simulink model "EPS Simulink Model"  (R2018b)
settings: Solver=VariableStepAuto  StartTime=0.0  StopTime=10.0  RelTol=1e-3
model workspace (MAT data in the model file):
  a = 4.4
  b = 2.25
settings Model: Creator=chaitu  LastModifiedBy=chaitu

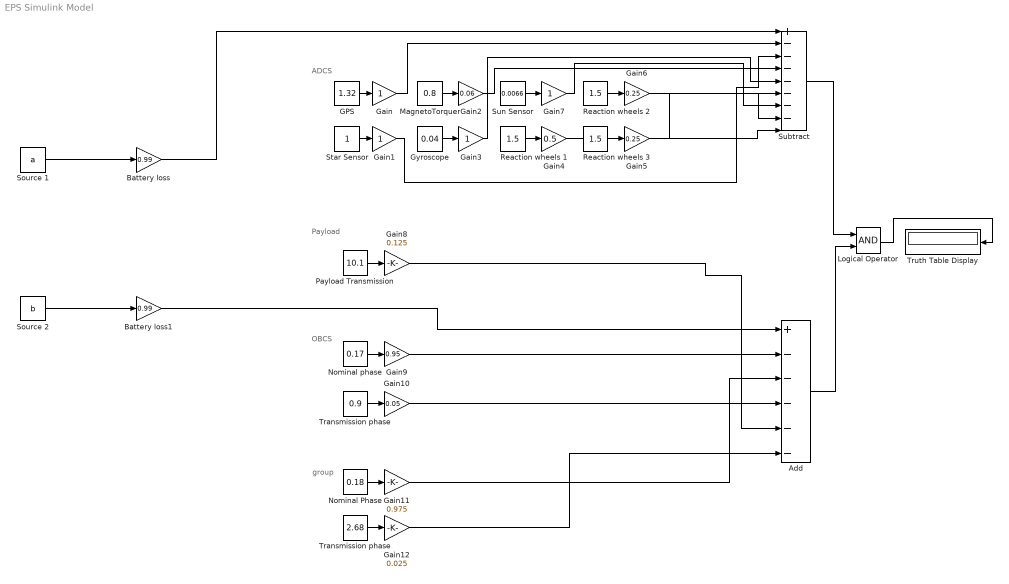
== system EPS Simulink Model ==
  note: group
  note: OBCS
  note: Payload
  note: ADCS
  Add : Sum  Inputs=+-----
  Battery loss : Gain  Gain=0.99
  Battery loss1 : Gain  Gain=0.99
  GPS : Constant  Value=1.32
  Gain{,1,3,7} (4 alike) : Gain
  Gain10 : Gain  Gain=0.05
  Gain11 : Gain  Gain=0.975
  Gain12 : Gain  Gain=0.025
  Gain2 : Gain  Gain=0.06
  Gain4 : Gain  Gain=0.5
  Gain5 : Gain  Gain=0.25
  Gain6 : Gain  Gain=0.25
  Gain8 : Gain  Gain=0.125
  Gain9 : Gain  Gain=0.95
  "Gyroscope " : Constant  Value=0.04
  Logical Operator : Logic  AllPortsSameDT=off  OutDataTypeStr=boolean
  MagnetoTorquer : Constant  Value=0.8
  "Nominal Phase " : Constant  Value=0.18
  "Nominal phase " : Constant  Value=0.17
  "Payload Transmission " : Constant  Value=10.1
  Reaction wheels 2 : Constant  Value=1.5
  Reaction wheels 3 : Constant  Value=1.5
  "Reaction wheels 1 " : Constant  Value=1.5
  "Source 1 " : Constant  Value=a
  "Source 2 " : Constant  Value=b
  "Star Sensor " : Constant
  Subtract : Sum  Inputs=+--------
  Sun Sensor : Constant  Value=0.0066
  Transmission phase : Constant  Value=2.68
  "Transmission phase " : Constant  Value=0.9
  "Truth Table Display " : Display
  wires:
  Battery loss/1 -> Subtract/1
  GPS/1 -> Gain/1
  "Star Sensor "/1 -> Gain1/1
  MagnetoTorquer/1 -> Gain2/1
  "Gyroscope "/1 -> Gain3/1
  "Reaction wheels 1 "/1 -> Gain4/1
  Reaction wheels 3/1 -> Gain5/1
  Reaction wheels 2/1 -> Gain6/1
  Sun Sensor/1 -> Gain7/1
  Gain/1 -> Subtract/2
  Gain1/1 -> Subtract/3
  Gain2/1 -> Subtract/4
  Gain3/1 -> Subtract/5
  Gain4/1 -> Subtract/6
  Gain7/1 -> Subtract/7
  Gain6/1 -> Subtract/8
  Gain5/1 -> Subtract/9
  "Payload Transmission "/1 -> Gain8/1
  "Nominal phase "/1 -> Gain9/1
  "Transmission phase "/1 -> Gain10/1
  "Nominal Phase "/1 -> Gain11/1
  Transmission phase/1 -> Gain12/1
  "Source 1 "/1 -> Battery loss/1
  Subtract/1 -> Logical Operator/1
  "Source 2 "/1 -> Battery loss1/1
  Gain9/1 -> Add/2
  Gain10/1 -> Add/4
  Gain11/1 -> Add/3
  Gain12/1 -> Add/6
  Gain8/1 -> Add/5
  Battery loss1/1 -> Add/1
  Add/1 -> Logical Operator/2
  Logical Operator/1 -> "Truth Table Display "/1
